simulink model "sine_wave"  (R2025b)
settings: Solver=FixedStepAuto  StartTime=0.0  StopTime=inf  RelTol=1e-3
settings Model: Creator=areeb-iqbal  LastModifiedBy=areeb-iqbal
settings SolverCC: AlgebraicLoopSolver=TrustRegion
settings DataIOCC: LimitDataPoints=on  SaveOutput=off  SaveTime=off
settings OptimizationCC: BooleanDataType=off  DefaultParameterBehavior=Inlined  LocalBlockOutputs=off  LifeSpan=inf
settings DebuggingCC: AlgebraicLoopMsg=error  SingleTaskRateTransMsg=error  UnconnectedInputMsg=warning  UnconnectedOutputMsg=warning  UnconnectedLineMsg=warning  AllowSymbolicDim=off  SFUnexpectedBacktrackingDiag=warning  SFNoUnconditionalDefaultTransitionDiag=warning  SFExecutionAtInitializationDiag=none  ArithmeticOperatorsInVariantConditions=warning
settings ModelReferenceCC: EnableRefExpFcnMdlSchedulingChecks=on
settings SFSimCC: SimUseLocalCustomCode=off  CustomCodeUndefinedFunction=UseInterfaceOnly
settings RTWCC: RTWUseLocalCustomCode=off  GPUComputeCapability=3.5
settings CodeAppCC: StateflowObjectComments=on
settings GRTTargetCC: TargetLangStandard=C89/C90 (ANSI)
settings ConfigComp: CovMetricSettings=dw  CovSaveCumulativeToWorkspaceVar=on  CovSaveSingleToWorkspaceVar=on  CovExternalEMLEnable=off  CovSFcnEnable=off

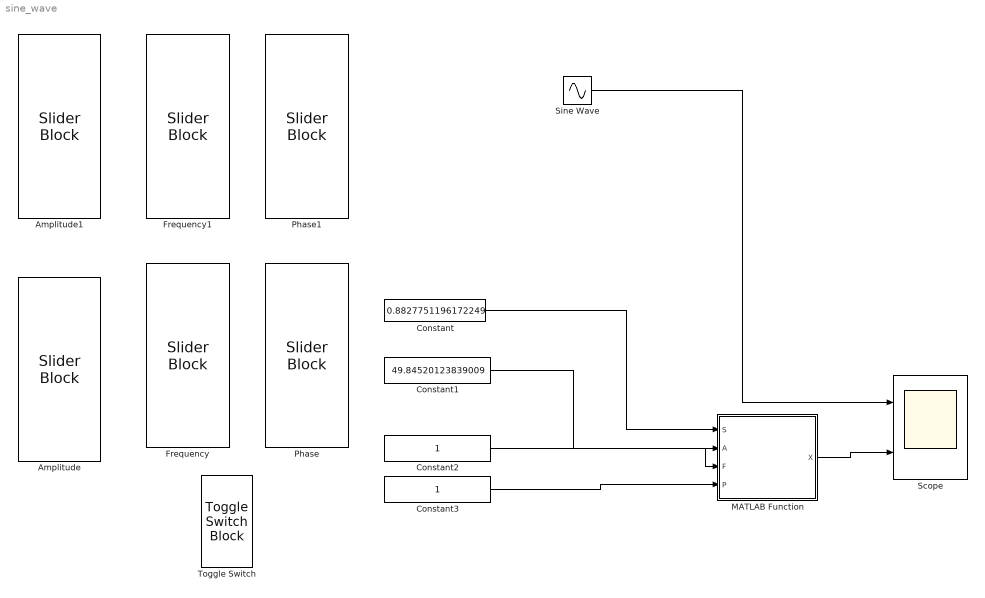
== system sine_wave ==
  Amplitude : SliderBlock  LabelPosition=Bottom  ScaleMax=1  TickInterval=0.25
  Amplitude1 : SliderBlock  LabelPosition=Bottom  ScaleMax=1  TickInterval=0.25
  Constant : Constant  Value=0.8827751196172249  OutMin=0  OutMax=1  OutDataTypeStr=double
  Constant1 : Constant  Value=49.84520123839009
  Constant2 : Constant
  Constant3 : Constant
  Frequency : SliderBlock  LabelPosition=Bottom  ScaleMax=200  TickInterval=50
  Frequency1 : SliderBlock  LabelPosition=Bottom  ScaleMax=200  TickInterval=50
  MATLAB Function : MATLAB Function  TreatAsAtomicUnit=on
  Phase : SliderBlock  LabelPosition=Bottom  ScaleMin=-1  ScaleMax=1  TickInterval=0.5
  Phase1 : SliderBlock  LabelPosition=Bottom  ScaleMin=-1  ScaleMax=1  TickInterval=0.5
  Scope : Scope  NumInputPorts=2
      settings: ActiveDisplayYMinimum=-16.95563340905106  ActiveDisplayYMaximum=13.965925129763789
  Sine Wave : Sin  Frequency=46.74922600619195  Phase=1  SampleTime=0
  Toggle Switch : ToggleSwitchBlock
  wires:
  Constant/1 -> MATLAB Function/1(S)
  Constant2/1 -> MATLAB Function/3(F)
  Constant1/1 -> MATLAB Function/2(A)
  Sine Wave/1 -> Scope/1
  MATLAB Function/1(X) -> Scope/2
  Constant3/1 -> MATLAB Function/4(P)

== matlab function sine_wave/MATLAB Function ==
  data: S input; A input; F input; P input; X output
function X = sine_gen_stateful(S, A, F, P)
%#codegen
persistent t0 first
Fs = 16000; N = 160;

if isempty(first)
    first = true; t0 = 0;
end

t = t0 + (0:N-1)/Fs;     % 1xN row

if first
    X = A .* sin(2*pi*F.*t + P*pi);
    first = false;
elseif S
    t0 = 0;
    t  = t0 + (0:N-1)/Fs;
    X  = A .* sin(2*pi*F.*t + P*pi);
else
    X = A .* sin(2*pi*F.*t);
    if t0 > 1
        t0 = t0 - (N/Fs);
    end
end

t0 = t0 + N/Fs;

% Ensure row vector for Simulink
X = reshape(X, 1, N);
end
